simulink model "Motor_control_simulation"  (R2018a)
settings: Solver=VariableStepAuto  StartTime=0.0  StopTime=20  RelTol=1e-3
settings Model: Creator=Hannes  LastModifiedBy=juli

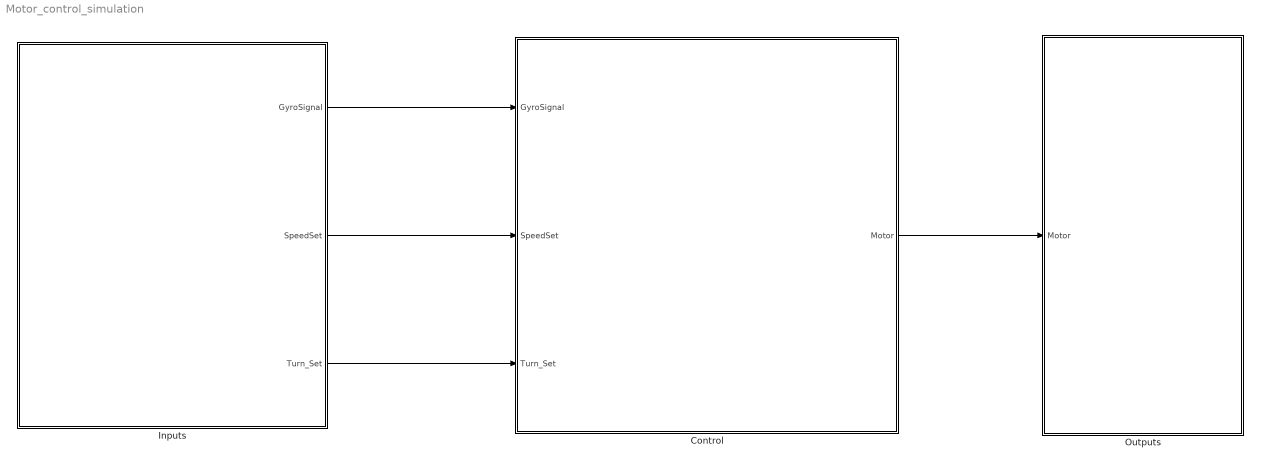
== system Motor_control_simulation ==
  Control : Subsystem
  Inputs : Subsystem
  "Outputs " : Subsystem
  wires:
  Inputs/1(GyroSignal) -> Control/1(GyroSignal)
  Inputs/3(Turn_Set) -> Control/3(Turn_Set)
  Inputs/2(SpeedSet) -> Control/2(SpeedSet)
  Control/1(Motor) -> "Outputs "/1(Motor)

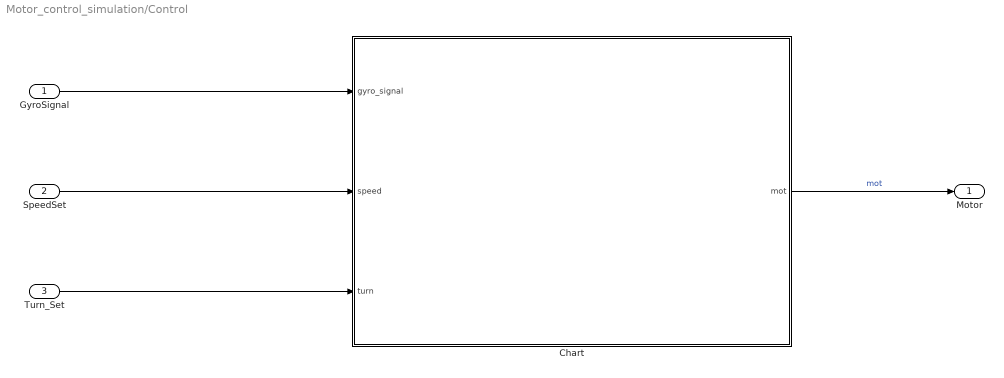
== system Motor_control_simulation/Control ==
  GyroSignal : Inport
  SpeedSet : Inport  Port=2
  Turn_Set : Inport  Port=3
  Chart : Stateflow chart  TreatAsAtomicUnit=on
  Motor : Outport
  wires:
  SpeedSet/1 -> Chart/2(speed)
  Turn_Set/1 -> Chart/3(turn)
  GyroSignal/1 -> Chart/1(gyro_signal)
  Chart/1(mot) -> Motor/1  "mot"

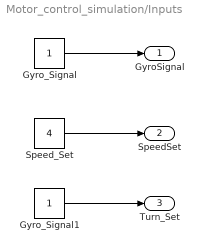
== system Motor_control_simulation/Inputs ==
  Gyro_Signal : Constant
  Gyro_Signal1 : Constant
  Speed_Set : Constant  Value=4
  GyroSignal : Outport
  SpeedSet : Outport  Port=2
  Turn_Set : Outport  Port=3
  wires:
  Speed_Set/1 -> SpeedSet/1
  Gyro_Signal1/1 -> Turn_Set/1
  Gyro_Signal/1 -> GyroSignal/1

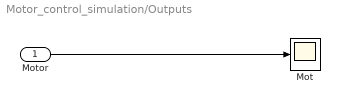
== system Motor_control_simulation/Outputs  ==
  Motor : Inport
  Mot : Scope
  wires:
  Motor/1 -> Mot/1

== stateflow chart Motor_control_simulation/Control/Chart ==
  settings: executeAtInitialization=1
  state Turn_Left
    entry: mot=-speed;
    during: mot=-speed;
    exit: mot=0;
  state Turn_Right
    entry: mot=speed;
    during: mot=speed;
    exit: mot=0;
  state Idle
    entry:mot=0;
    during:mot=0;
  Idle -> (junction 80) [order 2] : [turn>0]{curr_angle=gyro_signal;}
  (junction 80) -> Turn_Left [order 1] : [0<=(curr_angle+turn)<=360]{op=0}
  (junction 80) -> Turn_Left [order 2] : [curr_angle+turn<0]{op=360}
  Idle -> (junction 73) [order 1] : [turn<0]{curr_angle=gyro_signal;}
  (junction 73) -> Turn_Right [order 1] : [curr_angle+turn>360]{op=-360}
  (junction 73) -> Turn_Right [order 2] : [0<=(curr_angle+turn)<=360]{op=0}
  Turn_Right -> Idle : [(curr_angle+turn+op)-5<=gyro_signal || gyro_signal<=(curr_angle+turn+op)+5]{curr_angle=0}
  Turn_Left -> Idle : [(curr_angle+turn+op)-5<=gyro_signal || gyro_signal<=(curr_angle+turn+op)+5]{curr_angle=0}
  (default) -> Idle
  data: curr_angle local; gyro_signal input; speed input; turn input; mot output; op local
